simulink model "simulation"  (R2016b)
settings: Solver=FixedStepAuto  StartTime=0.0  StopTime=40.0  FixedStep=0.0001  RelTol=1e-3
settings Model: Creator=vanou  LastModifiedBy=vanou
settings OptimizationCC: BlockReduction=off  DefaultParameterBehavior=Inlined  BufferReuse=off

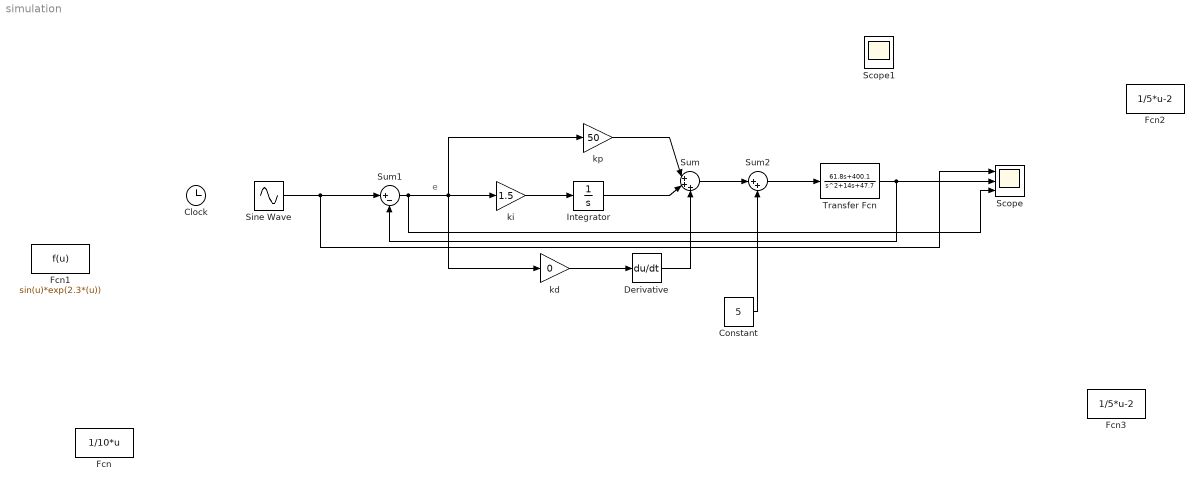
== system simulation ==
  note: e
  Clock : Clock
  Constant : Constant  Value=5
  Derivative : Derivative
  Fcn : Fcn  Expr=1/10*u
  Fcn1 : Fcn  Expr=sin(u)*exp(2.3*(u))
  Fcn2 : Fcn  Expr=1/5*u-2
  Fcn3 : Fcn  Expr=1/5*u-2
  Integrator : Integrator
  Scope : Scope  NumInputPorts=3
  Scope1 : Scope  NumInputPorts=2
  Sine Wave : Sin  SampleTime=0
  Sum : Sum  Inputs=|+++
  Sum1 : Sum  Inputs=|+-
  Sum2 : Sum  Inputs=|++
  Transfer Fcn : TransferFcn  Numerator="[61.8  400.1]"  Denominator="[1  14  47.7]"
  kd : Gain  Gain=0
  ki : Gain  Gain=1.5
  kp : Gain  Gain=50
  wires:
  kp/1 -> Sum/1
  Sum1/1 -> Scope/3, kd/1, ki/1, kp/1
  Transfer Fcn/1 -> Scope/2, Sum1/2
  ki/1 -> Integrator/1
  Integrator/1 -> Sum/2
  kd/1 -> Derivative/1
  Derivative/1 -> Sum/3
  Sine Wave/1 -> Scope/1, Sum1/1
  Sum/1 -> Sum2/1
  Sum2/1 -> Transfer Fcn/1
  Constant/1 -> Sum2/2
